simulink model "FuzzyPenduloInverso5x5"  (R2024b)
settings: Solver=VariableStepAuto  StartTime=0.0  StopTime=10.0  RelTol=1e-3
libraries: fuzblock x1
settings Model: Creator=david  LastModifiedBy=david

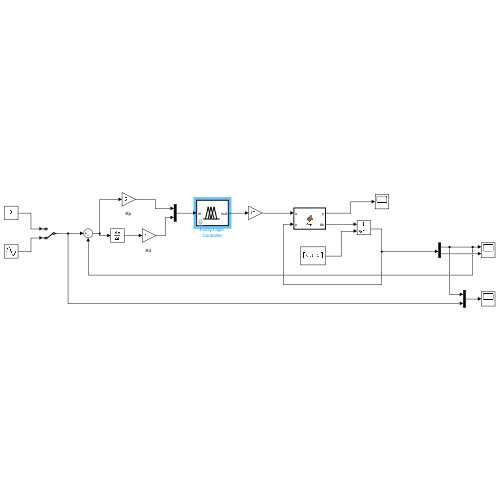
[thumbnail: Simulink's stored preview of the top-level diagram]
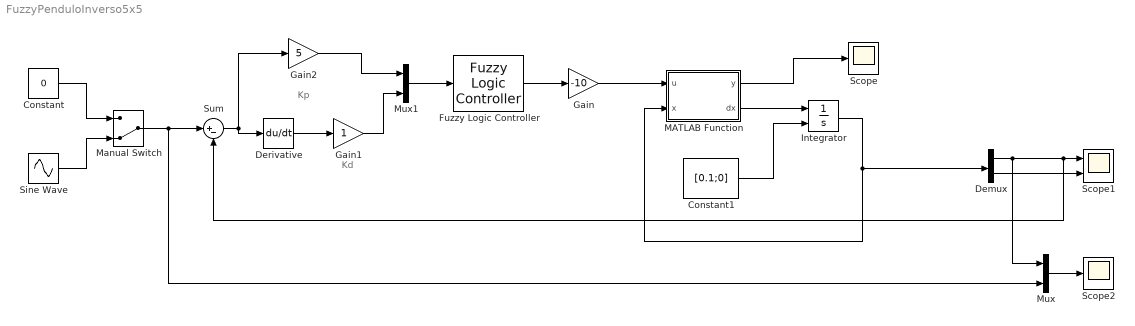
== system FuzzyPenduloInverso5x5 ==
  note: Kd
  note: Kp
  Constant : Constant  Value=0
  Constant1 : Constant  Value=[0.1;0]
  Demux : Demux  Outputs=2
  Derivative : Derivative
  Fuzzy Logic Controller : fuzblock/Fuzzy Logic  Controller  FIS='5x5man.fis'  OutputSampleNumber=101  DataType=double  FuzzifiedInputs=off  RuleFiringStrengths=off  RuleOutputs=off  AggregatedOutputs=off  SimulateUsing=Interpreted execution  OutOfRangeInputValueMessage=warning  NoRuleFiredMessage=warning  EmptyOutputFuzzySetMessage=warning
  Gain : Gain  Gain=-10
  Gain1 : Gain
  Gain2 : Gain  Gain=5
  Integrator : Integrator  InitialConditionSource=external
  MATLAB Function : MATLAB Function  TreatAsAtomicUnit=on
  Manual Switch : ManualSwitch  CurrentSetting=0
  Mux : Mux  Inputs=2
  Mux1 : Mux  Inputs=2
  Scope : Scope
  Scope1 : Scope  NumInputPorts=2
  Scope2 : Scope
  Sine Wave : Sin  Amplitude=0.25  Frequency=4  SampleTime=0
  Sum : Sum  Inputs=|+-
  wires:
  MATLAB Function/2(dx) -> Integrator/1
  Demux/2 -> Scope1/2
  Integrator/1 -> Demux/1, MATLAB Function/2(x)
  MATLAB Function/1(y) -> Scope/1
  Demux/1 -> Mux/1, Sum/2, Scope1/1
  Constant1/1 -> Integrator/2
  Gain/1 -> MATLAB Function/1(u)
  Fuzzy Logic Controller/1 -> Gain/1
  Sine Wave/1 -> Manual Switch/2
  Constant/1 -> Manual Switch/1
  Manual Switch/1 -> Mux/2, Sum/1
  Mux1/1 -> Fuzzy Logic Controller/1
  Derivative/1 -> Gain1/1
  Gain1/1 -> Mux1/2
  Sum/1 -> Gain2/1, Derivative/1
  Gain2/1 -> Mux1/1
  Mux/1 -> Scope2/1

== matlab function FuzzyPenduloInverso5x5/MATLAB Function ==
  data: y output; dx output; u input; x input
function [y, dx] = fcn(u, x)
g=9.81;
l=1;
m=1;
b=0.5;
I=m*l^2;

x1=x(1);
x2=x(2);
dx1=x2;
dx2= g/l * sin(x1) - b*l/I * x2 +u/I;

dx=[dx1, dx2];

y = u;
